simulink model "Sim_IntEnc_Deadzone_iqctest1"  (Simulink 7.3)
settings: Solver=ode45  StartTime=0.0  StopTime=20  RelTol=1e-3
settings Model: Creator=MD710  LastModifiedBy=MD710
settings DebuggingCC: SaveWithParameterizedLinksMsg=none  SolverPrmCheckMsg=none  MultiTaskDSMMsg=warning  MultiTaskCondExecSysMsg=none  FcnCallInpInsideContextMsg=Enable All  StrictBusMsg=None
settings HardwareCC: TargetHWDeviceType=32-bit Generic
settings RTWCC: IncludeERTFirstTime=on
settings GRTTargetCC: TargetFcnLib=ansi_tfl_tmw.mat

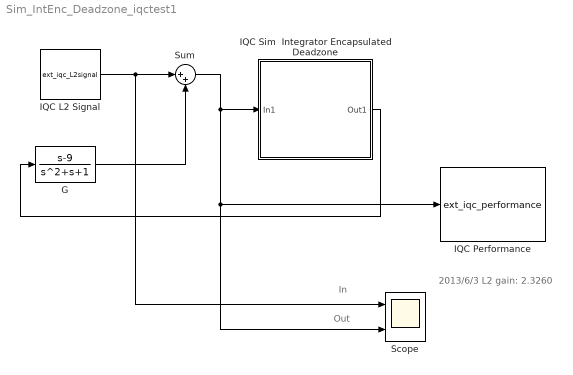
== system Sim_IntEnc_Deadzone_iqctest1 ==
  note: 2013/6/3 L2 gain: 2.3260
  note: In
  note: Out
  G : TransferFcn  Numerator=[1 -9]  Denominator=[1 1 1]
  IQC L2 Signal : M-S-Function  FunctionName=ext_iqc_L2signal  Parameters=sig_size,sam_time,sig_type,tru_time,sig_amp,sig_fre,user_cus  mask(IQC L2 signal(ver:0.1)){sig_size=1, sam_time=0, sig_type=Step, tru_time=5, sig_amp=2, sig_fre=1, user_cus='2*exp(3*t)'}
      mask prompts: sig_size "Signal Dimension:(Default: 1)"; sam_time "Sample Time:(Default: 0)"; sig_type "Signal Type:"; tru_time "Truncation Time:"; sig_amp "Maximum Amplitude:"; sig_fre "Frequency:"; user_cus "Custom:"
      mask help:
      | Important:
      | In IQC procedure step (as commond iqc_gain_tbx, the task is get
      | L2 gain value), regardless of the user to choose which option (ex sine...),
      | here regarded as generalized L2 signal.
      mask StyleString: edit,edit,popup(Step|Square wave|Sine wave|Custom|Random|External),edit,edit,edit,edit
      mask CallbackString: ||iqc_block_cho(gcb,'L2signal_type')||||
      mask TabNameString: Main,Main,Simulation,Simulation,Simulation,Simulation,Simulation
      mask Display: plot(0:0.1:10,[sin(0:0.1:6.2) zeros(1,38)])
  IQC Performance : M-S-Function  FunctionName=ext_iqc_performance  Parameters=imp_met,save_lin_com,isiqcbode,fre_ran,uselmitool,lmi_par  mask(IQC Performance(ver:0.1)){imp_met=Calculation and Simulation, save_lin_com=off, isiqcbode=off, fre_ran='', uselmitool=lmilab, lmi_par=''}
      mask prompts: imp_met "Implementation Methods"; save_lin_com "Save the Linear File and Command File"; isiqcbode "Display IQC Bode Figure"; fre_ran "Frequency Range:(Default: empty)"; uselmitool "LMI Tool:"; lmi_par "Parameter:(if empty use define)"
      mask help:
      | Important:
      | In IQC toolbox calculate step (as commond iqc_gain_tbx, the task is get
      | L2 gain value), regardless of the user to connect any signal input(Even if
      | not a signal), here regarded as generalized L2 signal.
      |
      | Example 1: setlmioptions('',[0 200 0 0 777])
      | the block parameter is
      | LMI Tool: lmilab
      | Parameter:
      |        [0 200 0 0 777]
      |
      | Example 2: setlmioptions('yalmip','solver','sdpt3','verbose',1)
      | the block parameter is
      | LMI Tool: yalmip
      | Parameter:
      |        {'solver',sdpt3','verbose',1}
      mask Help:
      | <a href="matlab:doc abst_init_iqc;">abst_init_iqc</a>
      | <a href="matlab:doc setlmioptions;">setlmioptions</a>
      | <a href="matlab:doc iqc_gain_tbx;">iqc_gain_tbx</a>
      mask StyleString: popup(Calculation and Simulation|Only Calculation|Only Simulation),checkbox,checkbox,edit,popup(lmilab|yalmip),edit
      mask CallbackString: iqc_block_cho(gcb,'performance_imp')||iqc_block_cho(gcb,'performance_bodefre')|||
      mask TabNameString: Main,Main,Main,Main,LMI,LMI
      mask Display: fprintf('In -> Out \n performance \n L2 gain:\n%4.4f',2.326);
  IQC Sim  Integrator Encapsulated Deadzone : Subsystem  mask(IQC Sim Integrator Encapsulated Deadzone(ver:0.1)){sta_dea=-1, end_dea=1, slo=0.3, iqc1=on, iqc1_pole=[1.8], iqc1_def_num_h=4, iqc1_out={'X'}, iqc2=off, iqc2_pole=[1], iqc2_def_num_h=0, iqc2_out='', iqc3=off, lis_rel=''}
      mask prompts: sta_dea "Start of Deadzone:"; end_dea "End of Deadzone:"; slo "Slope:"; iqc1 "iqc_dzn_e(Input,Pole,N,Slope)"; iqc1_pole "Pole:(Default: [1])"; iqc1_def_num_h "Defines Number of Terms in Expansion for H:(Default: 0)"; iqc1_out "Output Variable:(Default: empty)"; iqc2 "iqc_dzn_e_odd(Input,Pole,N,Slope)"; iqc2_pole "Pole:(Default: [1])"; iqc2_def_num_h "Defines Number of Terms in Expansion for H:(Default: 0)"; iqc2_out "Output Variable:(Default: empty)"; iqc3 "Custom IQC"; lis_rel "List of IQC Relationships:"
      mask Help:
      | <a href="matlab:doc iqc_dzn_e;">iqc_dzn_e</a>
      | <a href="matlab:doc iqc_dzn_e_odd;">iqc_dzn_e_odd</a>
      mask CallbackString: |||iqc_block_cho(gcb,'sim_intencdeadzone_iqc1')||||iqc_block_cho(gcb,'sim_intencdeadzone_iqc2')||||iqc_block_cho(gcb,'sim_intencdeadzone_iqc3')|
      mask TabNameString: Simulink Parameters,Simulink Parameters,Simulink Parameters,Procedure Parameters,Procedure Parameters,Procedure Parameters,Procedure Parameters,Procedure Parameters,Procedure Parameters,Procedure Parameters,Procedure Parameters,Procedure Parameters,Procedure Parameters
      mask Display: plot(0,0,100,100,[60,30,30,60,60],[90,90,60,60,90],[30,30,60,60,30],[40,10,10,40,40],[30,10,10,3,30],[25,25,76,76,76],[80,80,60],[72,25,25],[60,77],[76,76],[82,80,77,80,82,98],[76,72,76,80,76,76],[58,50,40,32],[88,76,76,63],[42,45,45,50],[15,17,34,36]);
  Scope : Scope  NumInputPorts=2
      settings: YMin=-1~-4e+016  YMax=1~3.5e+016
  Sum : Sum  Inputs=|++
  wires:
  IQC L2 Signal/1 -> Sum/1, Scope/1
  G/1 -> Sum/2
  Sum/1 -> IQC Performance/1, Scope/2, IQC Sim  Integrator Encapsulated Deadzone/1(In1)
  IQC Sim  Integrator Encapsulated Deadzone/1(Out1) -> G/1

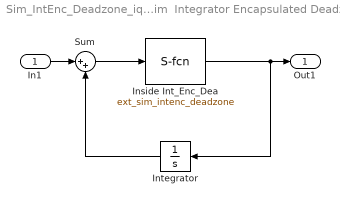
== system Sim_IntEnc_Deadzone_iqctest1/IQC Sim  Integrator Encapsulated Deadzone ==
  In1 : Inport
  Inside Int_Enc_Dea : M-S-Function  FunctionName=ext_sim_intenc_deadzone  Parameters=sta_dea,end_dea,slo,iqc1,iqc1_pole,iqc1_def_num_h,iqc1_out,iqc2,iqc2_pole,iqc2_def_num_h,iqc2_out,iqc3,lis_rel
  Integrator : Integrator
  Sum : Sum  Inputs=|++
  Out1 : Outport
  wires:
  In1/1 -> Sum/1
  Integrator/1 -> Sum/2
  Sum/1 -> Inside Int_Enc_Dea/1
  Inside Int_Enc_Dea/1 -> Integrator/1, Out1/1
